simulink model "PC_CONTROL_STATION"  (R2023b)
settings: Solver=FixedStepAuto  StartTime=0.0  StopTime=inf  RelTol=1e-3  EnableMultiTasking=on
InitFcn:
  | if RUN_MODE~=5
  |     % clear rpi;
  |     rpi = raspberrypi(CAR_IP, 'pi', 'LabControl');
  |     stopModel(rpi,'CAR_CONTROL_SYSTEM')
  |     while isModelRunning(rpi,'CAR_CONTROL_SYSTEM')
  |          stopModel(rpi,'CAR_CONTROL_SYSTEM')
  |     end
  |     runModel(rpi,'CAR_CONTROL_SYSTEM')
  |      while isModelRunning(rpi,'CAR_CONTROL_SYSTEM')==false
  |          runModel(rpi,'CAR_CONTROL_SYSTEM')
  |      end
  |      % clear rpi;
  | end
StopFcn:
  | if RUN_MODE~=5
  |    clear rpi;
  |    rpi = raspberrypi(CAR_IP, 'pi', 'LabControl');
  |    stopModel(rpi,'CAR_CONTROL_SYSTEM')
  |    while isModelRunning(rpi,'CAR_CONTROL_SYSTEM')
  |    end
  |    clear rpi;
  | end
model workspace (MAT data in the model file):
  SL_ROS_VariableLengthArrays_MaxSizes.CommonInfo.ArrayTruncateAction = 'EmitWarning'
  SL_ROS_VariableLengthArrays_MaxSizes.MsgTypeMap = containers.Map
  SL_ROS_VariableLengthArrays_MaxSizes.MsgTypeMap.serialization.keys = {'std_msgs/UInt8MultiArray'}
  SL_ROS_VariableLengthArrays_MaxSizes.MsgTypeMap.serialization.values{1}.PropertyName = 'data'
  SL_ROS_VariableLengthArrays_MaxSizes.MsgTypeMap.serialization.values{1}.DataType = 'uint8'
  SL_ROS_VariableLengthArrays_MaxSizes.MsgTypeMap.serialization.values{1}.MaxLength = 1400
  SL_ROS_VariableLengthArrays_MaxSizes.MsgTypeMap.serialization.uniformity = 0
  SL_ROS_VariableLengthArrays_MaxSizes.MsgTypeMap.serialization.keyType = 'char'
  SL_ROS_VariableLengthArrays_MaxSizes.MsgTypeMap.serialization.valueType = 'any'
values from neighbouring files (symbols this model uses):
  data = theClient.GetLastFrameOfData()    [FuncMotive.m]
undefined symbols (not defined in the file or in its folder): CONTROL, CONTROL_INI, data_SL_Info, MD25, MSG, SAMPLING_TIME, Standard_Devices, SYSID_INPUT, TCP_Protocol, UDP_Protocol
libraries: simulink x51, sldrtlib x46, dspsigattribs x7, ros2lib x3, ctrlSharedLib x2, aerolibanimutils x1
(part 1 of 8)
Description:
  | Packet Input/Output
  | 
  | The example model "sldrtex_packetio" shows how to transfer data through
  | UDP communication protocol using binary encoding. The model sends data
  | within one computer, from one UDP port to another. You can modify the
  | model to communicate between two computers by splitting this model
  | into its send and receive parts and running the models on two computers.
  | The yellow blocks are used to send the data, the blue blocks
  | are used to receive the data. Then, please enter the host names or
  | IP addresses of the two computers into the appropriate fields
  | in the Board Setup dialog.
  | 
  | How to run this model in Normal Mode:
  | 
  | 1) Double-click the orange button to switch to Normal Mode if needed.
  | 2) Start the real-time execution using Simulation->Run.
  | 
  | How to run this model in External Mode:
  | 
  | 1) Double-click the orange button to switch to External Mode if needed.
  | 2) Start the real-time execution using Simulation->Run. The model will automatically
  |    build, connect to Simulink in External Mode and start.
settings Model: SimulationMode=external  ExtModeTrigDuration=24000  Creator=The MathWorks, Inc.  LastModifiedBy=diego-ubuntu
settings SolverCC: AlgebraicLoopSolver=TrustRegion
settings DataIOCC: LimitDataPoints=on  SaveFormat=Array  SignalLoggingSaveFormat=ModelDataLogs  ReturnWorkspaceOutputs=off
settings OptimizationCC: EnhancedBackFolding=on  PassReuseOutputArgsThreshold=0  ExpressionDepthLimit=2147483647  InitFltsAndDblsToZero=on  EfficientMapNaN2IntZero=off  MaxStackSize=64  OptimizeBlockOrder=speed  DifferentSizesBufferReuse=on  OptimizationCustomize=off
settings DebuggingCC: MergeDetectMultiDrivingBlocksExec=none  SolverPrmCheckMsg=warning  ParameterTunabilityLossMsg=error  FcnCallInpInsideContextMsg=warning  UnconnectedInputMsg=warning  UnconnectedOutputMsg=warning  UnconnectedLineMsg=warning  AllowSymbolicDim=off  StateNameClashWarn=warning  SFUnexpectedBacktrackingDiag=warning  SFNoUnconditionalDefaultTransitionDiag=warning  SFExecutionAtInitializationDiag=none  ArithmeticOperatorsInVariantConditions=warning
settings HardwareCC: ProdBitPerLong=64  ProdHWDeviceType=Intel->x86-64 (Linux 64)
settings ModelReferenceCC: EnableRefExpFcnMdlSchedulingChecks=on  PropagateSignalLabelsOutOfModel=off
settings SFSimCC: SimUseLocalCustomCode=off  MATLABDynamicMemAlloc=off  CustomCodeUndefinedFunction=UseInterfaceOnly
settings RTWCC: Description=Simulink Desktop Real-Time  SystemTargetFile=sldrt.tlc  TemplateMakefile=sldrt.tmf  RTWUseLocalCustomCode=off  Toolchain=Colcon Tools  RTWCompilerOptimization=on  DLArmComputeVersion=19.05
settings CodeAppCC: ForceParamTrailComments=on  MaxIdLength=95  OperatorAnnotations=on
settings SimulinkDesktopRealTimeCC: TargetLibSuffix=_sldrt.a  TargetPreCompLibLocation=/usr/local/MATLAB/R2023b/toolbox/sldrt/lib/glnxa64  TargetLangStandard=C89/C90 (ANSI)
settings ConfigComp: CovMetricSettings=dsw  CovSaveCumulativeToWorkspaceVar=on  CovSaveSingleToWorkspaceVar=on  CovExternalEMLEnable=off

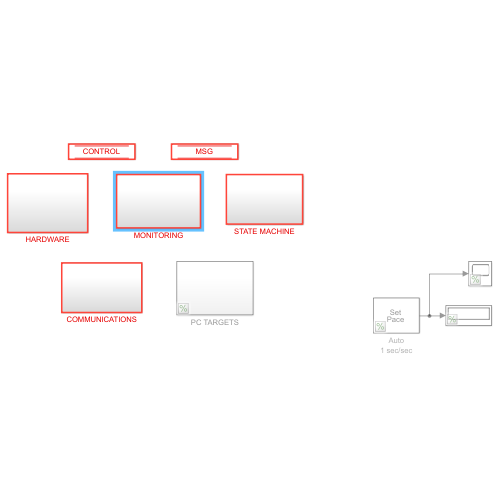
[thumbnail: Simulink's stored preview of the top-level diagram]
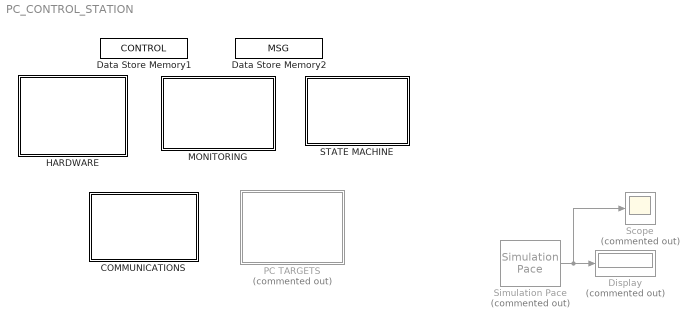
== system PC_CONTROL_STATION ==
  COMMUNICATIONS : Subsystem  Priority=40
      settings: RTWSystemCode=Nonreusable function  RTWFcnNameOpts=Use subsystem name  RTWFileNameOpts=Use subsystem name  FunctionWithSeparateData=on
  Data Store Memory1 : DataStoreMemory  Priority=2  DataStoreName=CONTROL  ReadBeforeWriteMsg=warning  WriteAfterWriteMsg=warning  WriteAfterReadMsg=warning  InitialValue=CONTROL_INI  ShowAdditionalParam=off  OutDataTypeStr=Bus: CONTROL_Bus
  Data Store Memory2 : DataStoreMemory  Priority=2  DataStoreName=MSG  ReadBeforeWriteMsg=warning  WriteAfterWriteMsg=warning  WriteAfterReadMsg=warning  InitialValue=MSG_INI  ShowAdditionalParam=off  OutDataTypeStr=Bus: MSG_Bus
  Display : Display  Commented=on
  HARDWARE : Subsystem  Priority=50  SystemSampleTime=SAMPLING_TIME
      settings: RTWSystemCode=Nonreusable function  RTWFcnNameOpts=Use subsystem name  RTWFileNameOpts=Use subsystem name  FunctionWithSeparateData=on
  MONITORING : Subsystem  Priority=1000
  PC TARGETS : Subsystem  Priority=5  Commented=on
  STATE MACHINE : Subsystem
  Scope : Scope  Commented=on
  Simulation Pace : aerolibanimutils/Simulation Pace  Commented=on  SimulationPace=1  SleepMode=Auto  OutputPaceError=on  SampleTime=CONTROL_INI.PARAM.COMM_SAMPLING_TIME
  wires:
  Simulation Pace/1 -> Scope/1, Display/1

== system PC_CONTROL_STATION/COMMUNICATIONS ==
  Compare To Zero1 : simulink/Logic and Bit Operations/Compare To Zero  relop=>  OutDataTypeStr=boolean
  Compare To Zero2 : simulink/Logic and Bit Operations/Compare To Zero  relop=>  OutDataTypeStr=boolean
  Compare To Zero3 : simulink/Logic and Bit Operations/Compare To Zero  relop=>  OutDataTypeStr=boolean
  Data Store Read1 : DataStoreRead  DataStoreName=MSG  SampleTime=CONTROL_INI.PARAM.COMM_SAMPLING_TIME  DataStoreElements=MSG.RX_BUFFER(1,1)  IndexOptions=Index vector (dialog)  Indices=1  OutputSizes=1
  Data Store Read2 : DataStoreRead  DataStoreName=CONTROL  DataStoreElements=CONTROL.STATE.CURRENT_STATUS_PC  IndexOptions=Index vector (dialog)  Indices=1  OutputSizes=1
  Data Store Read3 : DataStoreRead  DataStoreName=MSG  SampleTime=CONTROL_INI.PARAM.COMM_SAMPLING_TIME  DataStoreElements=MSG.TX_ID(1,1)  IndexOptions=Index vector (dialog)  Indices=1  OutputSizes=1
  Display1 : Display
  Display2 : Display
  Logical Operator1 : Logic  AllPortsSameDT=off  OutDataTypeStr=boolean
  MSG_RX : Subsystem  Priority=10
      settings: RTWSystemCode=Nonreusable function  FunctionWithSeparateData=on
  "MSG_TX " : Subsystem  Priority=10
      settings: RTWSystemCode=Nonreusable function  FunctionWithSeparateData=on
  wires:
  Data Store Read1/1 -> Compare To Zero1/1
  Data Store Read3/1 -> Compare To Zero2/1
  Compare To Zero2/1 -> "MSG_TX "/Enable, Display1/1
  Logical Operator1/1 -> MSG_RX/Enable, Display2/1
  Data Store Read2/1 -> Compare To Zero3/1
  Compare To Zero1/1 -> Logical Operator1/1
  Compare To Zero3/1 -> Logical Operator1/2

== system PC_CONTROL_STATION/HARDWARE ==
  ROS2_MONITORING : Subsystem
  RT_MONITORING : Subsystem  Commented=on

== system PC_CONTROL_STATION/MONITORING ==
  ADAPTIVE CONTROL STR : Subsystem  Commented=on
  FV COMPETITION: SCOPES : Subsystem  Commented=on  TreatAsAtomicUnit=on
      settings: MinAlgLoopOccurrences=on
  HARDWARE: SCOPES : Subsystem  Priority=1000  Commented=on
  NAV COMPETITION: SCOPES : Subsystem  Priority=20  Commented=on  TreatAsAtomicUnit=on
      settings: MinAlgLoopOccurrences=on
  PC: SCOPES : Subsystem
  SYSTEM IDENTIFICATION : Subsystem  Commented=on
      mask init:
      | %%%%%%%%%%%%%%%%%%%%%%%%%%%%%%%%%%%%%%%%%%%%%%%%%%%%%%
      | %%  STATE VARIABLE FILTER FOR SYSTEM IDENTIFICATION  %
      | %%%%%%%%%%%%%%%%%%%%%%%%%%%%%%%%%%%%%%%%%%%%%%%%%%%%%%
      | % Natural frequency (rad/s)
      | SVF_FREQ = 10;
      | % Factor defining band pass width
      | SVF_FACTOR = 5;
      | % FILTER ORDER/2
      | SVF_ORD = 2;
      | % Km/(Tm*Tf*s^2 + (Tm+Tf)*s + 1) = Km/Tm/Tf/(s^2 + (Tm+Tf)/Tm/Tf*s + 1/Tm/Tf)
      | % b0/(s^2 + a1*s + a0)
      | % D2y + a1*D1y + a0*y = b0*u
      | % D1y + a1*y + a0*I1y = b0*I1u
      | % D1yf = - a1*yf - a0*I1y + b0I1uf
      | %  -a1=-(Tm+Tf)/Tm/Tf / -a0=-1/Tm/Tf / b0=Km/Tm/Tf 
      | % Butterworh filter desig
      | [SVF_NUM,SVF_DEN]=butter(SVF_ORD,[SVF_FREQ/SVF_FACTOR SVF_FACTOR*SVF_FREQ],'s');
      | % Controlability canonical-form 
      | SVF_A = single([zeros(2*SVF_ORD-1,1) eye(2*SVF_ORD-1) ; -SVF_DEN(end:-1:2)]);
      | SVF_B = single([zeros(2*SVF_ORD-1,1) ; SVF_NUM(end-SVF_ORD)]);
      | % Sampling time
      | ts = 10e-3;
      | % Triangular hold
      | % x[k] = Ad*x[k-1] + B1d*u[k-1] + B2d*u[k]
      | % Ad = expm(A*ts)
      | % B1d = A\(Ad+inv(A)/ts-inv(A)*Ad/ts)*B;
      | % B2d = A\(inv(A)*Ad/ts-eye(2)-inv(A)/ts)*B;
      | SVF_Ad = expm(SVF_A*ts);
      | SVF_B1d = SVF_A\(SVF_Ad+inv(SVF_A)/ts-SVF_A\SVF_Ad/ts)*SVF_B;
      | SVF_B2d = SVF_A\(SVF_A\SVF_Ad/ts-eye(2*SVF_ORD)-inv(SVF_A)/ts)*SVF_B;

== system PC_CONTROL_STATION/PC TARGETS ==
  Compare To Constant4 : simulink/Logic and Bit Operations/Compare To Constant  relop=>  const=0  OutDataTypeStr=boolean
  Data Store Read9 : DataStoreRead  DataStoreName=CONTROL  SampleTime=SAMPLING_TIME  DataStoreElements=CONTROL.STATE.CONTROL_STATUS  IndexOptions=Index vector (dialog)  Indices=1  OutputSizes=1
  PC TARGETS : Subsystem  Priority=5  Commented=on  TreatAsAtomicUnit=on
      settings: MinAlgLoopOccurrences=on
  wires:
  Data Store Read9/1 -> Compare To Constant4/1
  Compare To Constant4/1 -> PC TARGETS/Enable

== system PC_CONTROL_STATION/STATE MACHINE ==
  Data Store Read2 : DataStoreRead  DataStoreName=MSG  SampleTime=CONTROL_INI.PARAM.COMM_SAMPLING_TIME  IndexOptions=Index vector (dialog)  Indices=1  OutputSizes=1
  Data Store Read7 : DataStoreRead  DataStoreName=CONTROL  SampleTime=CONTROL_INI.PARAM.COMM_SAMPLING_TIME  IndexOptions=Index vector (dialog)  Indices=1  OutputSizes=1
  Data Store Write1 : DataStoreWrite  DataStoreName=MSG  IndexOptions=Index vector (dialog)  Indices=1  OutputSizes=1
  Data Store Write3 : DataStoreWrite  DataStoreName=CONTROL  IndexOptions=Index vector (dialog)  Indices=1  OutputSizes=1
  Display : Display
  STATE MACHINE UPDATE : MATLAB Function  Priority=60  TreatAsAtomicUnit=on
  Scope : Scope
  wires:
  STATE MACHINE UPDATE/1(CONTROL) -> Data Store Write3/1
  Data Store Read7/1 -> STATE MACHINE UPDATE/1(CONTROL_IN)
  Data Store Read2/1 -> STATE MACHINE UPDATE/2(MSG_IN)
  STATE MACHINE UPDATE/2(MSG) -> Data Store Write1/1
  STATE MACHINE UPDATE/3(DATA_DIFF) -> Scope/1, Display/1

== system PC_CONTROL_STATION/COMMUNICATIONS/MSG_RX ==
  Enable : EnablePort
  Data Store Read : DataStoreRead  DataStoreName=MSG  SampleTime=CONTROL_INI.PARAM.COMM_SAMPLING_TIME  IndexOptions=Index vector (dialog)  Indices=1  OutputSizes=1
  Data Store Read2 : DataStoreRead  DataStoreName=CONTROL  SampleTime=CONTROL_INI.PARAM.COMM_SAMPLING_TIME  IndexOptions=Index vector (dialog)  Indices=1  OutputSizes=1
  Data Store Write1 : DataStoreWrite  DataStoreName=MSG  SampleTime=CONTROL_INI.PARAM.COMM_SAMPLING_TIME  IndexOptions=Index vector (dialog)  Indices=1  OutputSizes=1
  Data Store Write2 : DataStoreWrite  DataStoreName=CONTROL  SampleTime=CONTROL_INI.PARAM.COMM_SAMPLING_TIME  IndexOptions=Index vector (dialog)  Indices=1  OutputSizes=1
  MSG DECODER : MATLAB Function  Priority=20  TreatAsAtomicUnit=on
  wires:
  MSG DECODER/1(MSG) -> Data Store Write1/1
  Data Store Read/1 -> MSG DECODER/1(MSG_IN)
  MSG DECODER/2(CONTROL) -> Data Store Write2/1
  Data Store Read2/1 -> MSG DECODER/2(CONTROL_IN)

== system PC_CONTROL_STATION/COMMUNICATIONS/MSG_TX  ==
  Enable : EnablePort
  Data Store Read : DataStoreRead  DataStoreName=MSG  SampleTime=CONTROL_INI.PARAM.COMM_SAMPLING_TIME  IndexOptions=Index vector (dialog)  Indices=1  OutputSizes=1
  Data Store Read6 : DataStoreRead  DataStoreName=CONTROL  SampleTime=CONTROL_INI.PARAM.COMM_SAMPLING_TIME  IndexOptions=Index vector (dialog)  Indices=1  OutputSizes=1
  Data Store Write1 : DataStoreWrite  DataStoreName=MSG  SampleTime=CONTROL_INI.PARAM.COMM_SAMPLING_TIME  IndexOptions=Index vector (dialog)  Indices=1  OutputSizes=1
  MSG CODER : MATLAB Function  Priority=20  TreatAsAtomicUnit=on
  wires:
  Data Store Read/1 -> MSG CODER/1(MSG_IN)
  MSG CODER/1(MSG) -> Data Store Write1/1
  Data Store Read6/1 -> MSG CODER/2(CONTROL)

== system PC_CONTROL_STATION/HARDWARE/ROS2_MONITORING ==
  Compare To Zero : simulink/Logic and Bit Operations/Compare To Zero  relop=>  OutDataTypeStr=boolean
  Data Store Read : DataStoreRead  DataStoreName=MSG  SampleTime=CONTROL_INI.PARAM.COMM_SAMPLING_TIME  DataStoreElements=MSG.TX_BUFFER(1,1)  IndexOptions=Index vector (dialog)  Indices=1  OutputSizes=1
  MSG_RX : Subsystem  Priority=10
      settings: RTWSystemCode=Nonreusable function  FunctionWithSeparateData=on
  "MSG_TX " : Subsystem  Priority=10
      settings: RTWSystemCode=Nonreusable function  FunctionWithSeparateData=on
  wires:
  Compare To Zero/1 -> "MSG_TX "/Enable
  Data Store Read/1 -> Compare To Zero/1

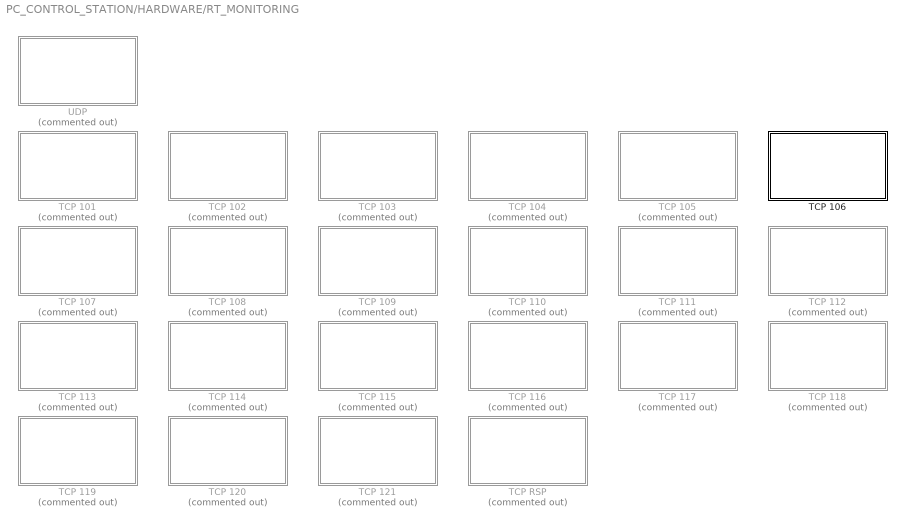
== system PC_CONTROL_STATION/HARDWARE/RT_MONITORING ==
  TCP 101 : Subsystem  Commented=on
  TCP 102 : Subsystem  Commented=on
  TCP 103 : Subsystem  Commented=on
  TCP 104 : Subsystem  Commented=on
  TCP 105 : Subsystem  Commented=on
  TCP 106 : Subsystem
  TCP 107 : Subsystem  Commented=on
  TCP 108 : Subsystem  Commented=on
  TCP 109 : Subsystem  Commented=on
  TCP 110 : Subsystem  Commented=on
  TCP 111 : Subsystem  Commented=on
  TCP 112 : Subsystem  Commented=on
  TCP 113 : Subsystem  Commented=on
  TCP 114 : Subsystem  Commented=on
  TCP 115 : Subsystem  Commented=on
  TCP 116 : Subsystem  Commented=on
  TCP 117 : Subsystem  Commented=on
  TCP 118 : Subsystem  Commented=on
  TCP 119 : Subsystem  Commented=on
  TCP 120 : Subsystem  Commented=on
  TCP 121 : Subsystem  Commented=on
  TCP RSP : Subsystem  Commented=on
  UDP : Subsystem  Commented=on

== system PC_CONTROL_STATION/MONITORING/ADAPTIVE CONTROL STR ==
  Data Store Read : DataStoreRead  DataStoreName=CONTROL  SampleTime=SAMPLING_TIME  DataStoreElements=CONTROL.TARGET.FORWARD_VEL_REF#CONTROL.INPUT.FORWARD_VEL#CONTROL.OUTPUT.MOTOR_VOLT_CD(1,1)#CONTROL.PARAM.VEL_GAIN#CONTROL.PARAM.VEL_GAIN_EST#CONTROL.PARAM.VEL_TIME_CONSTANT#CONTROL.PARAM.VEL_TIME_CONSTANT_EST#CONTROL.PARAM.FILT_TIME_CONSTANT_ACT#CONTROL.PARAM.FILT_TIME_CONSTANT_EST#CONTROL.PARAM.FORWARD_VEL_PID.K#CONTROL.PARAM.FV_PI_STR_K#CONTROL.PARAM.FORWARD_VEL_PID.Ti#CONTROL.PARAM.FV_PI_STR_Ti#CONTROL.PARAM.FORWARD_VEL_PID.b#CONTROL.PARAM.FV_PI_STR_b#CONTROL.PARAM.ADPT_FLAG  IndexOptions=Index vector (dialog)  Indices=1  OutputSizes=1
  Mux{1..7} (7 alike) : Mux  Inputs=2
  SCOPE_STR : Scope  NumInputPorts=9
  wires:
  Mux4/1 -> SCOPE_STR/1
  Data Store Read/1 -> Mux4/1
  Data Store Read/2 -> Mux4/2
  Data Store Read/3 -> SCOPE_STR/2
  Mux1/1 -> SCOPE_STR/3
  Data Store Read/4 -> Mux1/1
  Data Store Read/5 -> Mux1/2
  Mux2/1 -> SCOPE_STR/4
  Data Store Read/6 -> Mux2/1
  Data Store Read/7 -> Mux2/2
  Mux3/1 -> SCOPE_STR/5
  Data Store Read/8 -> Mux3/1
  Data Store Read/9 -> Mux3/2
  Mux5/1 -> SCOPE_STR/6
  Data Store Read/10 -> Mux5/1
  Data Store Read/11 -> Mux5/2
  Data Store Read/12 -> Mux6/1
  Data Store Read/13 -> Mux6/2
  Mux6/1 -> SCOPE_STR/7
  Mux7/1 -> SCOPE_STR/8
  Data Store Read/14 -> Mux7/1
  Data Store Read/15 -> Mux7/2
  Data Store Read/16 -> SCOPE_STR/9

== system PC_CONTROL_STATION/MONITORING/FV COMPETITION: SCOPES ==
  Data Store Read1 : DataStoreRead  DataStoreName=CONTROL  SampleTime=SAMPLING_TIME  DataStoreElements=CONTROL.TARGET.FORWARD_VEL_REF#CONTROL.INPUT.FORWARD_VEL#CONTROL.OUTPUT.MOTOR_VOLT_CD(1,1)#CONTROL.STATE.COMP_IAE  IndexOptions=Index vector (dialog)  Indices=1  OutputSizes=1
  Display : Display
  FV COMPETITION SCOPE: SIM : Scope  NumInputPorts=3
  Mux6 : Mux  Inputs=2
  wires:
  Mux6/1 -> FV COMPETITION SCOPE: SIM/1
  Data Store Read1/1 -> Mux6/1
  Data Store Read1/2 -> Mux6/2
  Data Store Read1/3 -> FV COMPETITION SCOPE: SIM/2
  Data Store Read1/4 -> Display/1, FV COMPETITION SCOPE: SIM/3

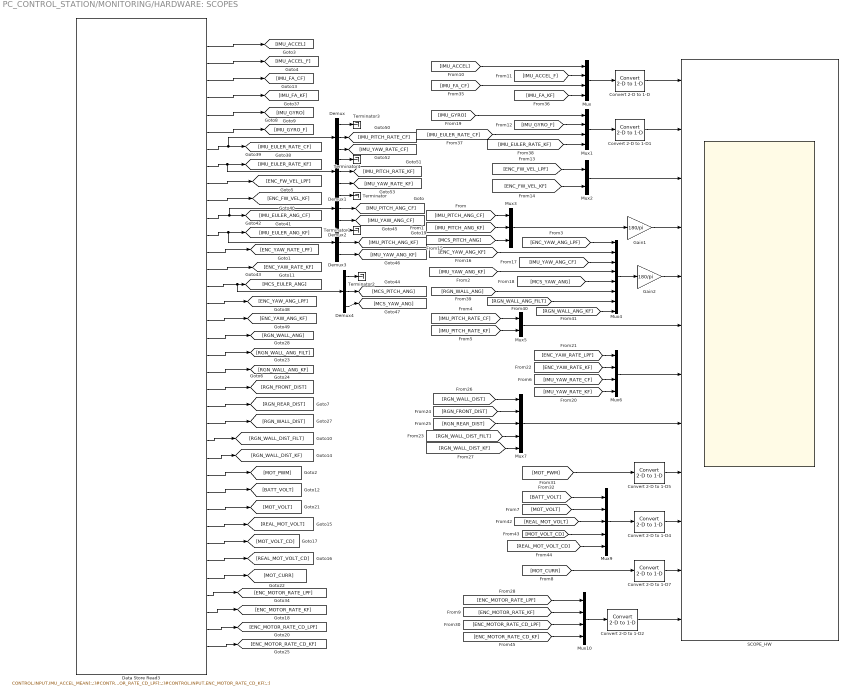
== system PC_CONTROL_STATION/MONITORING/HARDWARE: SCOPES ==
  Convert 2-D to 1-D{,1..2,4..5,7} (6 alike) : dspsigattribs/Convert 2-D to 1-D
  Data Store Read3 : DataStoreRead  DataStoreName=CONTROL  SampleTime=CONTROL_INI.PARAM.COMM_SAMPLING_TIME  DataStoreElements=CONTROL.INPUT.IMU_ACCEL_MEAN(:,:)#CONTROL.INPUT.IMU_ACCEL_MEAN_FILT(:,:)#CONTROL.INPUT.IMU_FORWARD_ACCEL_CF#CONTROL.INPUT.IMU_FORWARD_ACCEL_KF#CONTROL.INPUT.IMU_GYRO_MEAN(:,:)#CONTROL.INPUT.IMU_GYRO_MEAN_FILT(:,:)#CONTROL.INPUT.IMU_EULER_RATE_CF(:,:)#CONTROL.INPUT.IMU_EULER_RATE_KF(:,:)#CONTROL.INPUT.ENC_FORWARD_VEL_LPF#CONTROL.INPUT.ENC_FORWARD_VEL_KF#CONTROL.INPUT.IMU_EULER_ANG_CF(:,:)#CONTROL.INPUT.IMU_EULER_ANG_KF(:,:)#CONTROL.INPUT.ENC_YAW_RATE_LPF#CONTROL.INPUT.ENC_YAW_RATE_KF#CONTROL.INPUT.MCS_EULER_ANG(:,:)#CONTROL.INPUT.ENC_YAW_ANG_LPF#CONTROL.INPUT.ENC_YAW_ANG_KF#CONTROL.INPUT.RANGE_WALL_ANG#CONTROL.INPUT.WALL_ANG_FILT#CONTROL.INPUT.WALL_ANG_KF#CONTROL.INPUT.RANGE_FRONT_DIST#CONTROL.INPUT.RANGE_REAR_DIST#CONTROL.INPUT.RANGE_WALL_DIST#CONTROL.INPUT.WALL_DIST_FILT#CONTROL.INPUT.WALL_DIST_KF#CONTROL.OUTPUT.MOTOR_PWM(:,:)#CONTROL.INPUT.BATTERY_VOLT#CONTROL.OUTPUT.MOTOR_VOLT(:,:)#CONTROL.OUTPUT.REAL_MOTOR_VOLT(:,:)#CONTROL.OUTPUT.MOTOR_VOLT_CD(:,:)#CONTROL.OUTPUT.REAL_MOTOR_VOLT_CD(:,:)#CONTROL.INPUT.MOTOR_CURRENT(:,:)#CONTROL.INPUT.ENC_MOTOR_RATE_LPF(:,:)#CONTROL.INPUT.ENC_MOTOR_RATE_KF(:,:)#CONTROL.INPUT.ENC_MOTOR_RATE_CD_LPF(:,:)#CONTROL.INPUT.ENC_MOTOR_RATE_CD_KF(:,:)  IndexOptions=Index vector (dialog)  Indices=1  OutputSizes=1
  Demux{,1..4} (5 alike) : Demux  Outputs=3
  Gain1 : Gain  Gain=180/pi
  Gain2 : Gain  Gain=180/pi
  Mux{,1,6,10} (4 alike) : Mux
  Mux2 : Mux  Inputs=2
  Mux3 : Mux  Inputs=3
  Mux4 : Mux  Inputs=8
  Mux5 : Mux  Inputs=2
  Mux7 : Mux  Inputs=5
  Mux9 : Mux  Inputs=5
  SCOPE_HW : Scope  NumInputPorts=12
  Terminator{,1..4} (5 alike) : Terminator
  wires:
  [MOT_CURR] -> Convert 2-D to 1-D7/1
  Convert 2-D to 1-D/1 -> SCOPE_HW/1
  Convert 2-D to 1-D1/1 -> SCOPE_HW/2
  Mux2/1 -> SCOPE_HW/3
  [IMU_ACCEL] -> Mux/1
  Mux/1 -> Convert 2-D to 1-D/1
  [IMU_ACCEL_F] -> Mux/2
  [ENC_FW_VEL_LPF] -> Mux2/1
  [ENC_FW_VEL_KF] -> Mux2/2
  [IMU_PITCH_ANG_CF] -> Mux3/1
  [IMU_PITCH_ANG_KF] -> Mux3/2
  Mux3/1 -> Gain1/1
  Gain1/1 -> SCOPE_HW/4
  Mux4/1 -> Gain2/1
  Gain2/1 -> SCOPE_HW/5
  Mux5/1 -> SCOPE_HW/6
  [IMU_PITCH_RATE_CF] -> Mux5/1
  [IMU_PITCH_RATE_KF] -> Mux5/2
  Mux6/1 -> SCOPE_HW/7
  Mux7/1 -> SCOPE_HW/8
  [RGN_WALL_DIST] -> Mux7/1
  [RGN_FRONT_DIST] -> Mux7/2
  [RGN_REAR_DIST] -> Mux7/3
  Mux9/1 -> Convert 2-D to 1-D4/1
  [MOT_VOLT] -> Mux9/2
  [BATT_VOLT] -> Mux9/1
  [MOT_PWM] -> Convert 2-D to 1-D5/1
  Convert 2-D to 1-D5/1 -> SCOPE_HW/9
  Convert 2-D to 1-D4/1 -> SCOPE_HW/10
  Convert 2-D to 1-D7/1 -> SCOPE_HW/11
  Data Store Read3/1 -> [IMU_ACCEL]
  Data Store Read3/2 -> [IMU_ACCEL_F]
  [ENC_MOTOR_RATE_KF] -> Mux10/2
  Mux10/1 -> Convert 2-D to 1-D2/1
  [ENC_MOTOR_RATE_LPF] -> Mux10/1
  Data Store Read3/32 -> [MOT_CURR]
  Data Store Read3/33 -> [ENC_MOTOR_RATE_LPF]
  Data Store Read3/34 -> [ENC_MOTOR_RATE_KF]
  Data Store Read3/5 -> [IMU_GYRO]
  Data Store Read3/6 -> [IMU_GYRO_F]
  Data Store Read3/3 -> [IMU_FA_CF]
  Data Store Read3/4 -> [IMU_FA_KF]
  [IMU_FA_CF] -> Mux/3
  [IMU_FA_KF] -> Mux/4
  Data Store Read3/7 -> Demux/1, [IMU_EULER_RATE_CF]
  Data Store Read3/8 -> Demux1/1, [IMU_EULER_RATE_KF]
  Mux1/1 -> Convert 2-D to 1-D1/1
  [IMU_GYRO] -> Mux1/1
  [IMU_GYRO_F] -> Mux1/2
  [IMU_EULER_RATE_CF] -> Mux1/3
  [IMU_EULER_RATE_KF] -> Mux1/4
  Data Store Read3/9 -> [ENC_FW_VEL_LPF]
  Data Store Read3/10 -> [ENC_FW_VEL_KF]
  Data Store Read3/11 -> Demux2/1, [IMU_EULER_ANG_CF]
  Data Store Read3/12 -> Demux3/1, [IMU_EULER_ANG_KF]
  Demux2/2 -> [IMU_PITCH_ANG_CF]
  Demux3/2 -> [IMU_PITCH_ANG_KF]
  Demux4/2 -> [MCS_PITCH_ANG]
  [MCS_PITCH_ANG] -> Mux3/3
  Demux2/3 -> [IMU_YAW_ANG_CF]
  Demux3/3 -> [IMU_YAW_ANG_KF]
  Demux2/1 -> Terminator/1
  Demux3/1 -> Terminator1/1
  Demux4/3 -> [MCS_YAW_ANG]
  Demux4/1 -> Terminator2/1
  [ENC_YAW_ANG_LPF] -> Mux4/1
  [ENC_YAW_ANG_KF] -> Mux4/2
  [IMU_YAW_ANG_CF] -> Mux4/3
  [IMU_YAW_ANG_KF] -> Mux4/4
  [MCS_YAW_ANG] -> Mux4/5
  [RGN_WALL_ANG] -> Mux4/6
  [RGN_WALL_ANG_FILT] -> Mux4/7
  [RGN_WALL_ANG_KF] -> Mux4/8
  Demux/2 -> [IMU_PITCH_RATE_CF]
  Demux1/2 -> [IMU_PITCH_RATE_KF]
  Demux/1 -> Terminator3/1
  Demux1/1 -> Terminator4/1
  Demux/3 -> [IMU_YAW_RATE_CF]
  Demux1/3 -> [IMU_YAW_RATE_KF]
  Data Store Read3/14 -> [ENC_YAW_RATE_KF]
  Data Store Read3/15 -> Demux4/1, [MCS_EULER_ANG]
  Data Store Read3/16 -> [ENC_YAW_ANG_LPF]
  Data Store Read3/17 -> [ENC_YAW_ANG_KF]
  Data Store Read3/18 -> [RGN_WALL_ANG]
  Data Store Read3/19 -> [RGN_WALL_ANG_FILT]
  Data Store Read3/20 -> [RGN_WALL_ANG_KF]
  Data Store Read3/13 -> [ENC_YAW_RATE_LPF]
  Data Store Read3/21 -> [RGN_FRONT_DIST]
  Data Store Read3/22 -> [RGN_REAR_DIST]
  Data Store Read3/23 -> [RGN_WALL_DIST]
  Data Store Read3/24 -> [RGN_WALL_DIST_FILT]
  Data Store Read3/25 -> [RGN_WALL_DIST_KF]
  [RGN_WALL_DIST_FILT] -> Mux7/4
  [RGN_WALL_DIST_KF] -> Mux7/5
  Data Store Read3/26 -> [MOT_PWM]
  Data Store Read3/27 -> [BATT_VOLT]
  Data Store Read3/28 -> [MOT_VOLT]
  Data Store Read3/29 -> [REAL_MOT_VOLT]
  Data Store Read3/31 -> [REAL_MOT_VOLT_CD]
  Data Store Read3/30 -> [MOT_VOLT_CD]
  [REAL_MOT_VOLT_CD] -> Mux9/5
  [REAL_MOT_VOLT] -> Mux9/3
  [MOT_VOLT_CD] -> Mux9/4
  Data Store Read3/35 -> [ENC_MOTOR_RATE_CD_LPF]
  Data Store Read3/36 -> [ENC_MOTOR_RATE_CD_KF]
  [ENC_MOTOR_RATE_CD_LPF] -> Mux10/3
  [ENC_MOTOR_RATE_CD_KF] -> Mux10/4
  Convert 2-D to 1-D2/1 -> SCOPE_HW/12
  [IMU_YAW_RATE_CF] -> Mux6/3
  [IMU_YAW_RATE_KF] -> Mux6/4
  [ENC_YAW_RATE_LPF] -> Mux6/1
  [ENC_YAW_RATE_KF] -> Mux6/2

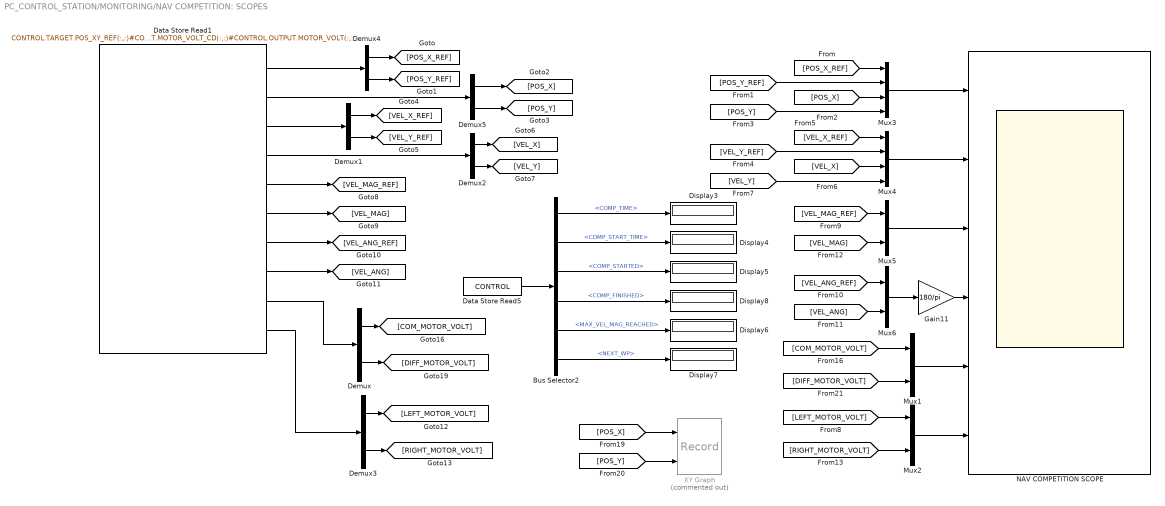
== system PC_CONTROL_STATION/MONITORING/NAV COMPETITION: SCOPES ==
  Bus Selector2 : BusSelector  OutputSignals=STATE.COMP_TIME,STATE.COMP_START_TIME,STATE.COMP_STARTED,STATE.COMP_FINISHED,STATE.MAX_VEL_MAG_REACHED,STATE.NEXT_WP
  Data Store Read1 : DataStoreRead  DataStoreName=CONTROL  SampleTime=SAMPLING_TIME  DataStoreElements=CONTROL.TARGET.POS_XY_REF(:,:)#CONTROL.INPUT.EARTH_POS(1:2,1)#CONTROL.TARGET.VEL_XY_REF(:,:)#CONTROL.INPUT.EARTH_VEL(1:2,1)#CONTROL.TARGET.NAV_REF(1,1)#CONTROL.INPUT.NAV_MO(1,1)#CONTROL.TARGET.NAV_REF(2,1)#CONTROL.INPUT.NAV_MO(2,1)#CONTROL.OUTPUT.MOTOR_VOLT_CD(:,:)#CONTROL.OUTPUT.MOTOR_VOLT(:,:)  IndexOptions=Index vector (dialog)  Indices=1  OutputSizes=1
  Data Store Read5 : DataStoreRead  DataStoreName=CONTROL  SampleTime=SAMPLING_TIME  IndexOptions=Index vector (dialog)  Indices=1  OutputSizes=1
  Demux{,1..5} (6 alike) : Demux  Outputs=2
  Display{3..8} (6 alike) : Display
  Gain11 : Gain  Gain=180/pi
  Mux{1..2,5..6} (4 alike) : Mux  Inputs=2
  Mux3 : Mux
  Mux4 : Mux
  NAV COMPETITION SCOPE : Scope  NumInputPorts=6
  XY Graph : Record  Commented=on  FileSettingsInternal="{\"entries\":[{\"content\":{\"excelSettings\":{\"content\":{},\"type\":\"Streamout.ExcelSettings\"}},\"type\":\"Streamout.FileSettingStorage\",\"uuid\":\"\"}],\"packageUris\":[\"http:\\/\\/schema.mathworks.com\\/mf0\\/streamout_blocks\\/R2020a\"],\"version\":\"1.0\"}"  Layout=[1 1]  SignalsInternal="{\"entries\":[{\"content\":{\"signals\":[{\"content\":{\"blockPath\":[],\"dimensions\":[1],\"domain\":\"\",\"lineColor\":\"#a2142f\",\"plots\":[ 1 ],\"port\":1,\"signalID\":1,\"signalName\":\"XY Graph:1\"},\"type\":\"RecordBlkView.Signal\",\"uuid\":\"\"},{\"content\":{\"blockPath\":[],\"dimensions\":[1],\"domain\":\"\",\"lineColor\":\"#139fff\",\"plots\":[ 1 ],\"port\":2,\"signalID\":2,\"signalName\":\"XY Graph:2\"},\"type\":\"RecordBlkView.Signal\",\"uuid\":\"\"}]},\"type\":\"RecordBlkView.InputSignals\",\"uuid\":\"\"}],\"packageUris\":[\"http:\\/\\/schema.mathworks.com\\/mf0\\/streamout_blocks\\/R2020a\"],\"version\":\"1.0\"}"  VisualizationBindings="{\"xyplotplugin\":{\"info\":[{\"series\":[{\"bindingParametersList\":[{\"parameter\":\"X-Axis\",\"signalID\":1,\"signalName\":\"XY Graph:1\"},{\"parameter\":\"Y-Axis\",\"signalID\":2,\"signalName\":\"XY Graph:2\"}],\"seriesID\":0}],\"subplotID\":1}]}}"  CompatibilityTag=XY  st=SAMPLING_TIME
  wires:
  Bus Selector2/1 -> Display3/1  "<COMP_TIME>"
  Bus Selector2/4 -> Display8/1  "<COMP_FINISHED>"
  Bus Selector2/3 -> Display5/1  "<COMP_STARTED>"
  Bus Selector2/2 -> Display4/1  "<COMP_START_TIME>"
  Bus Selector2/6 -> Display7/1  "<NEXT_WP>"
  Mux4/1 -> NAV COMPETITION SCOPE/2
  Bus Selector2/5 -> Display6/1  "<MAX_VEL_MAG_REACHED>"
  Gain11/1 -> NAV COMPETITION SCOPE/4
  Mux3/1 -> NAV COMPETITION SCOPE/1
  Mux6/1 -> Gain11/1
  Mux5/1 -> NAV COMPETITION SCOPE/3
  Data Store Read5/1 -> Bus Selector2/1
  Demux4/1 -> [POS_X_REF]
  Demux4/2 -> [POS_Y_REF]
  Demux5/1 -> [POS_X]
  Demux5/2 -> [POS_Y]
  [POS_X_REF] -> Mux3/1
  [VEL_X_REF] -> Mux4/1
  [VEL_Y] -> Mux4/4
  [VEL_MAG_REF] -> Mux5/1
  [VEL_MAG] -> Mux5/2
  [VEL_ANG_REF] -> Mux6/1
  [VEL_ANG] -> Mux6/2
  Data Store Read1/9 -> Demux/1
  [POS_X] -> XY Graph/1
  [POS_Y] -> XY Graph/2
  Demux1/1 -> [VEL_X_REF]
  Demux1/2 -> [VEL_Y_REF]
  Demux2/2 -> [VEL_Y]
  Demux2/1 -> [VEL_X]
  Data Store Read1/1 -> Demux4/1
  Data Store Read1/2 -> Demux5/1
  Data Store Read1/3 -> Demux1/1
  Data Store Read1/4 -> Demux2/1
  Data Store Read1/5 -> [VEL_MAG_REF]
  Data Store Read1/6 -> [VEL_MAG]
  Data Store Read1/7 -> [VEL_ANG_REF]
  Data Store Read1/8 -> [VEL_ANG]
  Demux/1 -> [COM_MOTOR_VOLT]
  Demux/2 -> [DIFF_MOTOR_VOLT]
  [COM_MOTOR_VOLT] -> Mux1/1
  [DIFF_MOTOR_VOLT] -> Mux1/2
  Mux1/1 -> NAV COMPETITION SCOPE/5
  Mux2/1 -> NAV COMPETITION SCOPE/6
  [RIGHT_MOTOR_VOLT] -> Mux2/2
  [LEFT_MOTOR_VOLT] -> Mux2/1
  Data Store Read1/10 -> Demux3/1
  Demux3/1 -> [LEFT_MOTOR_VOLT]
  Demux3/2 -> [RIGHT_MOTOR_VOLT]
  [POS_Y_REF] -> Mux3/2
  [POS_X] -> Mux3/3
  [POS_Y] -> Mux3/4
  [VEL_Y_REF] -> Mux4/2
  [VEL_X] -> Mux4/3

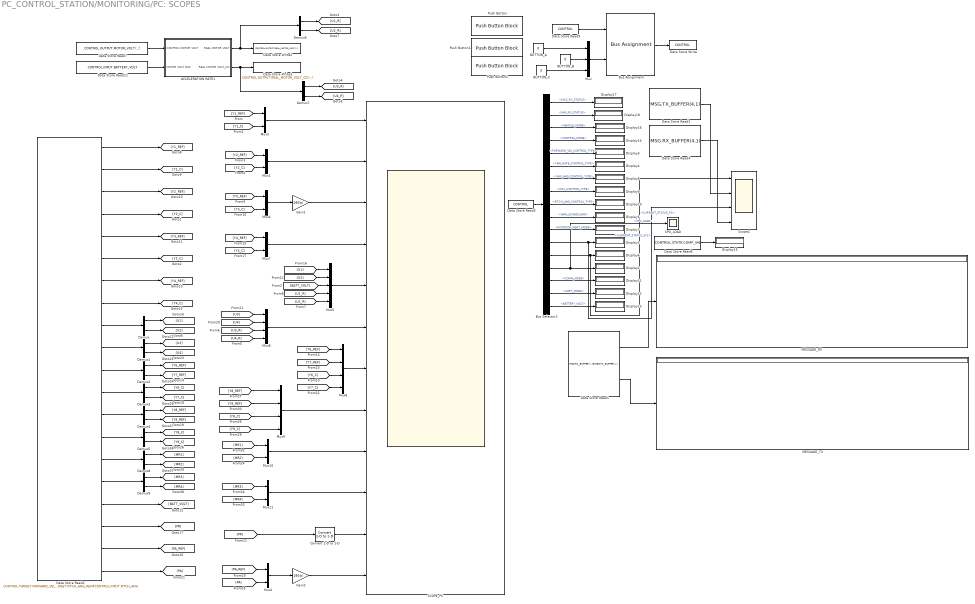
== system PC_CONTROL_STATION/MONITORING/PC: SCOPES ==
  ACCELERATION RATE1 : Subsystem  Priority=50  TreatAsAtomicUnit=on
      settings: MinAlgLoopOccurrences=on
  BUTTON_A : Constant  Value=0  OutDataTypeStr=uint8  SampleTime=CONTROL_INI.PARAM.COMM_SAMPLING_TIME
  BUTTON_B : Constant  Value=0  OutDataTypeStr=uint8  SampleTime=CONTROL_INI.PARAM.COMM_SAMPLING_TIME
  BUTTON_C : Constant  Value=0  OutDataTypeStr=uint8  SampleTime=CONTROL_INI.PARAM.COMM_SAMPLING_TIME
  Bus Assignment : BusAssignment  Priority=40  AssignedSignals=STATE.PC_BUTTONS
  Bus Selector2 : BusSelector  OutputSignals=STATE.MCS_RX_STATUS,STATE.NAV_RX_STATUS,STATE.VEHICLE_MODE,STATE.CONTROL_MODE,STATE.FORWARD_VEL_CONTROL_TYPE,STATE.YAW_RATE_CONTROL_TYPE,STATE.YAW_ANG_CONTROL_TYPE,STATE.WFL_CONTROL_TYPE,STATE.PITCH_ANG_CONTROL_TYPE,STATE.GAIN_SCHEDULING,STATE.ROTATION_MSRT_MODE,STATE.CURRENT_STATUS_SYS,STATE.CURRENT_STATUS_PC,STATE.CPU_LOAD,STATE.COMM_MODE,STATE.UART_MODE,INPUT.BATTERY_VOLT
  CPU_LOAD : Scope
  Convert 2-D to 1-D : dspsigattribs/Convert 2-D to 1-D
  Data Store Read1 : DataStoreRead  DataStoreName=MSG  SampleTime=CONTROL_INI.PARAM.COMM_SAMPLING_TIME  DataStoreElements=MSG.RX_BUFFER(:,:)#MSG.TX_BUFFER(:,:)  IndexOptions=Index vector (dialog)  Indices=1  OutputSizes=1
  Data Store Read11 : DataStoreRead  DataStoreName=CONTROL  SampleTime=CONTROL_INI.PARAM.COMM_SAMPLING_TIME  DataStoreElements=CONTROL.INPUT.BATTERY_VOLT  IndexOptions=Index vector (dialog)  Indices=1  OutputSizes=1
  Data Store Read2 : DataStoreRead  DataStoreName=CONTROL  SampleTime=CONTROL_INI.PARAM.COMM_SAMPLING_TIME  DataStoreElements=CONTROL.TARGET.FORWARD_VEL_REF#CONTROL.INPUT.FORWARD_VEL#CONTROL.TARGET.YAW_RATE_REF#CONTROL.INPUT.YAW_RATE#CONTROL.TARGET.YAW_ANG_REF#CONTROL.INPUT.YAW_ANG#CONTROL.TARGET.WALL_DIST_REF#CONTROL.INPUT.WALL_DIST#CONTROL.OUTPUT.MOTOR_VOLT(:,:)#CONTROL.OUTPUT.MOTOR_VOLT_CD(:,:)#CONTROL.TARGET.POS_XY_REF(:,:)#CONTROL.INPUT.EARTH_POS(1:2,1)#CONTROL.TARGET.VEL_XY_REF(:,:)#CONTROL.INPUT.EARTH_VEL(1:2,1)#CONTROL.INPUT.MOTOR_RATE(:,:)#CONTROL.INPUT.MOTOR_RATE_CD(:,:)#CONTROL.INPUT.BATTERY_VOLT#CONTROL.INPUT.PITCH_RATE#CONTROL.TARGET.PITCH_ANG_REF#CONTROL.INPUT.PITCH_ANG  IndexOptions=Index vector (dialog)  Indices=1  OutputSizes=1
  Data Store Read3 : DataStoreRead  DataStoreName=MSG  SampleTime=CONTROL_INI.PARAM.COMM_SAMPLING_TIME  DataStoreElements=MSG.TX_BUFFER(4,1)  IndexOptions=Index vector (dialog)  Indices=1  OutputSizes=1
  Data Store Read4 : DataStoreRead  DataStoreName=MSG  SampleTime=CONTROL_INI.PARAM.COMM_SAMPLING_TIME  DataStoreElements=MSG.RX_BUFFER(4,1)  IndexOptions=Index vector (dialog)  Indices=1  OutputSizes=1
  Data Store Read5 : DataStoreRead  DataStoreName=CONTROL  SampleTime=CONTROL_INI.PARAM.COMM_SAMPLING_TIME  IndexOptions=Index vector (dialog)  Indices=1  OutputSizes=1
  Data Store Read6 : DataStoreRead  DataStoreName=CONTROL  SampleTime=CONTROL_INI.PARAM.COMM_SAMPLING_TIME  DataStoreElements=CONTROL.STATE.COMP_IAE  IndexOptions=Index vector (dialog)  Indices=1  OutputSizes=1
  Data Store Read7 : DataStoreRead  DataStoreName=CONTROL  SampleTime=CONTROL_INI.PARAM.COMM_SAMPLING_TIME  DataStoreElements=CONTROL.OUTPUT.MOTOR_VOLT(:,:)  IndexOptions=Index vector (dialog)  Indices=1  OutputSizes=1
  Data Store Read9 : DataStoreRead  DataStoreName=CONTROL  SampleTime=CONTROL_INI.PARAM.COMM_SAMPLING_TIME  IndexOptions=Index vector (dialog)  Indices=1  OutputSizes=1
  Data Store Write : DataStoreWrite  DataStoreName=CONTROL  IndexOptions=Index vector (dialog)  Indices=1  OutputSizes=1
  Data Store Write2 : DataStoreWrite  DataStoreName=CONTROL  DataStoreElements=CONTROL.OUTPUT.REAL_MOTOR_VOLT(:,:)  IndexOptions=Index vector (dialog)  Indices=1  OutputSizes=1
  Data Store Write3 : DataStoreWrite  DataStoreName=CONTROL  DataStoreElements=CONTROL.OUTPUT.REAL_MOTOR_VOLT_CD(:,:)  IndexOptions=Index vector (dialog)  Indices=1  OutputSizes=1
  Demux{,1..9} (10 alike) : Demux  Outputs=2
  Display{1..18} (18 alike) : Display
  Gain1 : Gain  Gain=180/pi
  Gain2 : Gain  Gain=180/pi
  MESSAGE_RX : Display
  MESSAGE_TX : Display
  Mux : Mux  Inputs=3
  Mux{1..4,7,10..11} (7 alike) : Mux  Inputs=2
  Mux5 : Mux  Inputs=5
  Mux6 : Mux
  Mux8 : Mux
  Mux9 : Mux
  Push Button : PushButtonBlock  ButtonText=BUTTON A  OffValue=0.000000
  Push Button1 : PushButtonBlock  ButtonText=BUTTON B  OffValue=0.000000
  Push Button2 : PushButtonBlock  ButtonText=BUTTON C  OffValue=0.000000
  SCOPE_PC : Scope  NumInputPorts=12
  Scope2 : Scope  NumInputPorts=4
  wires:
  Data Store Read5/1 -> Bus Selector2/1
  Bus Selector2/11 -> Display7/1  "<ROTATION_MSRT_MODE>"
  Data Store Read1/1 -> MESSAGE_RX/1
  Bus Selector2/10 -> Display5/1  "<GAIN_SCHEDULING>"
  Bus Selector2/12 -> Display1/1, Scope2/3  "<CURRENT_STATUS_SYS>"
  Bus Selector2/14 -> CPU_LOAD/1, Display2/1  "<CPU_LOAD>"
  Data Store Read1/2 -> MESSAGE_TX/1
  Mux/1 -> Bus Assignment/2
  Data Store Read9/1 -> Bus Assignment/1
  Bus Assignment/1 -> Data Store Write/1
  BUTTON_C/1 -> Mux/3
  BUTTON_B/1 -> Mux/2
  BUTTON_A/1 -> Mux/1
  Bus Selector2/13 -> Scope2/1, Display6/1  "<CURRENT_STATUS_PC>"
  Data Store Read3/1 -> Scope2/2
  Data Store Read4/1 -> Scope2/4
  Demux8/2 -> [MR2]
  Demux9/1 -> [MR3]
  Data Store Read2/16 -> Demux9/1
  Data Store Read2/15 -> Demux8/1
  Data Store Read2/2 -> [Y1_C]
  Data Store Read2/7 -> [Y4_REF]
  Demux4/1 -> [Y8_REF]
  Demux5/1 -> [Y8_C]
  Demux3/1 -> [Y6_C]
  Demux2/1 -> [Y6_REF]
  Demux1/1 -> [U3]
  Demux3/2 -> [Y7_C]
  Demux5/2 -> [Y9_C]
  Demux4/2 -> [Y9_REF]
  Demux2/2 -> [Y7_REF]
  Data Store Read2/5 -> [Y3_REF]
  Demux/2 -> [U2]
  Data Store Read2/1 -> [Y1_REF]
  Demux1/2 -> [U4]
  Demux8/1 -> [MR1]
  Data Store Read2/4 -> [Y2_C]
  Data Store Read2/6 -> [Y3_C]
  Demux9/2 -> [MR4]
  Data Store Read2/3 -> [Y2_REF]
  Data Store Read2/8 -> [Y4_C]
  Demux/1 -> [U1]
  [MR1] -> Mux10/1
  [MR4] -> Mux11/2
  Gain1/1 -> SCOPE_PC/3
  Mux10/1 -> SCOPE_PC/9
  Mux8/1 -> SCOPE_PC/6
  Mux6/1 -> SCOPE_PC/7
  Mux5/1 -> SCOPE_PC/5
  Mux7/1 -> SCOPE_PC/4
  [MR3] -> Mux11/1
  [U4] -> Mux8/2
  Mux11/1 -> SCOPE_PC/10
  [Y8_REF] -> Mux9/1
  [Y4_REF] -> Mux7/1
  [Y3_C] -> Mux4/2
  [Y4_C] -> Mux7/2
  [U1] -> Mux5/1
  Mux9/1 -> SCOPE_PC/8
  [Y1_C] -> Mux3/2
  [U3] -> Mux8/1
  [U2] -> Mux5/2
  [Y2_C] -> Mux1/2
  [Y2_REF] -> Mux1/1
  Mux3/1 -> SCOPE_PC/1
  [Y1_REF] -> Mux3/1
  [MR2] -> Mux10/2
  Mux4/1 -> Gain1/1
  Mux1/1 -> SCOPE_PC/2
  [Y3_REF] -> Mux4/1
  [Y6_REF] -> Mux6/1
  [Y7_C] -> Mux6/4
  Data Store Read2/9 -> Demux/1
  Data Store Read2/10 -> Demux1/1
  Data Store Read2/11 -> Demux2/1
  Data Store Read2/12 -> Demux3/1
  Data Store Read2/13 -> Demux4/1
  Data Store Read2/14 -> Demux5/1
  Bus Selector2/15 -> Display11/1  "<COMM_MODE>"
  Bus Selector2/16 -> Display12/1  "<UART_MODE>"
  Bus Selector2/17 -> Display13/1  "<BATTERY_VOLT>"
  Data Store Read2/17 -> [BATT_VOLT]
  [BATT_VOLT] -> Mux5/3
  [U3_R] -> Mux8/3
  [U4_R] -> Mux8/4
  [U1_R] -> Mux5/4
  [U2_R] -> Mux5/5
  ACCELERATION RATE1/1(REAL MOTOR VOLT) -> Demux6/1, Data Store Write2/1
  Demux7/1 -> [U3_R]
  Demux7/2 -> [U4_R]
  Demux6/2 -> [U2_R]
  Demux6/1 -> [U1_R]
  ACCELERATION RATE1/2(REAL MOTOR VOLT_CD) -> Demux7/1, Data Store Write3/1
  Data Store Read6/1 -> Display15/1
  Data Store Read2/20 -> [PA]
  Data Store Read2/19 -> [PA_REF]
  Data Store Read2/18 -> [PR]
  Mux2/1 -> Gain2/1
  [PA] -> Mux2/2
  [PA_REF] -> Mux2/1
  Gain2/1 -> SCOPE_PC/12
  [PR] -> Convert 2-D to 1-D/1
  Bus Selector2/4 -> Display14/1  "<CONTROL_MODE>"
  Bus Selector2/5 -> Display3/1  "<FORWARD_VEL_CONTROL_TYPE>"
  Bus Selector2/6 -> Display4/1  "<YAW_RATE_CONTROL_TYPE>"
  Bus Selector2/7 -> Display8/1  "<YAW_ANG_CONTROL_TYPE>"
  Bus Selector2/8 -> Display9/1  "<WFL_CONTROL_TYPE>"
  Bus Selector2/9 -> Display10/1  "<PITCH_ANG_CONTROL_TYPE>"
  Bus Selector2/3 -> Display16/1  "<VEHICLE_MODE>"
  [Y9_REF] -> Mux9/2
  [Y8_C] -> Mux9/3
  [Y9_C] -> Mux9/4
  [Y7_REF] -> Mux6/2
  [Y6_C] -> Mux6/3
  Convert 2-D to 1-D/1 -> SCOPE_PC/11
  Bus Selector2/1 -> Display17/1  "<MCS_RX_STATUS>"
  Data Store Read11/1 -> ACCELERATION RATE1/2(MOTOR VOLT MAX)
  Data Store Read7/1 -> ACCELERATION RATE1/1(CONTROL MOTOR VOLT)
  Bus Selector2/2 -> Display18/1  "<NAV_RX_STATUS>"

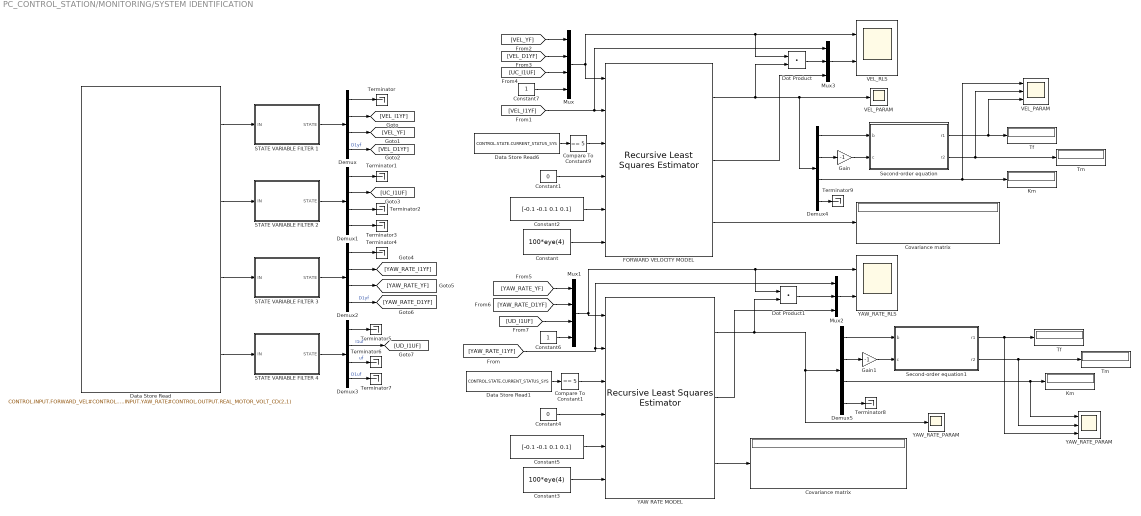
== system PC_CONTROL_STATION/MONITORING/SYSTEM IDENTIFICATION ==
  Compare To Constant1 : simulink/Logic and Bit Operations/Compare To Constant  relop===  const=5  OutDataTypeStr=boolean
  Compare To Constant9 : simulink/Logic and Bit Operations/Compare To Constant  relop===  const=5  OutDataTypeStr=boolean
  Constant : Constant  Value=100*eye(4)  SampleTime=SAMPLING_TIME
  Constant1 : Constant  Value=0  SampleTime=SAMPLING_TIME
  Constant2 : Constant  Value=[-0.1 -0.1 0.1 0.1]  SampleTime=SAMPLING_TIME
  Constant3 : Constant  Value=100*eye(4)  SampleTime=SAMPLING_TIME
  Constant4 : Constant  Value=0  SampleTime=SAMPLING_TIME
  Constant5 : Constant  Value=[-0.1 -0.1 0.1 0.1]  SampleTime=SAMPLING_TIME
  Constant6 : Constant  OutDataTypeStr=double  SampleTime=SAMPLING_TIME
  Constant7 : Constant  OutDataTypeStr=double  SampleTime=SAMPLING_TIME
  Covariance matrix : Display
  "Covariance matrix " : Display
  Data Store Read : DataStoreRead  DataStoreName=CONTROL  SampleTime=SAMPLING_TIME  DataStoreElements=CONTROL.INPUT.FORWARD_VEL#CONTROL.OUTPUT.REAL_MOTOR_VOLT_CD(1,1)#CONTROL.INPUT.YAW_RATE#CONTROL.OUTPUT.REAL_MOTOR_VOLT_CD(2,1)  IndexOptions=Index vector (dialog)  Indices=1  OutputSizes=1
  Data Store Read1 : DataStoreRead  DataStoreName=CONTROL  SampleTime=SAMPLING_TIME  DataStoreElements=CONTROL.STATE.CURRENT_STATUS_SYS  IndexOptions=Index vector (dialog)  Indices=1  OutputSizes=1
  Data Store Read6 : DataStoreRead  DataStoreName=CONTROL  SampleTime=SAMPLING_TIME  DataStoreElements=CONTROL.STATE.CURRENT_STATUS_SYS  IndexOptions=Index vector (dialog)  Indices=1  OutputSizes=1
  Demux{,1..5} (6 alike) : Demux
  Dot Product : DotProduct  OutDataTypeStr=Inherit: Inherit via internal rule
  Dot Product1 : DotProduct  OutDataTypeStr=Inherit: Inherit via internal rule
  FORWARD VELOCITY MODEL : ctrlSharedLib/Recursive Least Squares Estimator  InitialEstimateSource=External  InitialParameterData=4  P0=1e4  InitialRegressors=0  InitialOutputs=0  History=Infinite  WindowLength=200  EstimationMethod=Forgetting Factor  AdaptationParameter=0.999  HasTimeVaryingAdaptationParameter=off  NormalizationBias=eps  OutputError=on  OutputP=on  AddEnablePort=on  ExternalReset=Rising  InputProcessing=Sample-based  Ts=SAMPLING_TIME
  Gain : Gain  Gain=-1
  Gain1 : Gain  Gain=-1
  Km : Display
  "Km " : Display
  Mux : Mux
  Mux1 : Mux
  Mux2 : Mux  Inputs=3
  Mux3 : Mux  Inputs=3
  STATE VARIABLE FILTER 1 : Subsystem
  STATE VARIABLE FILTER 2 : Subsystem
  STATE VARIABLE FILTER 3 : Subsystem
  STATE VARIABLE FILTER 4 : Subsystem
  Second-order equation : MATLAB Function  TreatAsAtomicUnit=on
  Second-order equation1 : MATLAB Function  TreatAsAtomicUnit=on
  Terminator{,1..9} (10 alike) : Terminator
  Tf : Display
  "Tf " : Display
  Tm : Display
  "Tm " : Display
  VEL_PARAM : Scope
  "VEL_PARAM " : Scope  NumInputPorts=3
  VEL_RLS : Scope  NumInputPorts=2
  YAW RATE MODEL : ctrlSharedLib/Recursive Least Squares Estimator  InitialEstimateSource=External  InitialParameterData=4  P0=1e4  InitialRegressors=0  InitialOutputs=0  History=Infinite  WindowLength=200  EstimationMethod=Forgetting Factor  AdaptationParameter=0.999  HasTimeVaryingAdaptationParameter=off  NormalizationBias=eps  OutputError=on  OutputP=on  AddEnablePort=on  ExternalReset=Rising  InputProcessing=Sample-based  Ts=SAMPLING_TIME
  YAW_RATE_PARAM : Scope
  "YAW_RATE_PARAM " : Scope  NumInputPorts=3
  YAW_RATE_RLS : Scope  NumInputPorts=2
  wires:
  STATE VARIABLE FILTER 1/1(STATE) -> Demux/1
  Demux/1 -> Terminator/1
  STATE VARIABLE FILTER 2/1(STATE) -> Demux1/1
  Demux1/1 -> Terminator1/1
  Demux1/3 -> Terminator2/1
  Demux1/4 -> Terminator3/1
  Constant/1 -> FORWARD VELOCITY MODEL/6
  Constant1/1 -> FORWARD VELOCITY MODEL/4
  Constant2/1 -> FORWARD VELOCITY MODEL/5
  Constant5/1 -> YAW RATE MODEL/5
  Constant4/1 -> YAW RATE MODEL/4
  Constant3/1 -> YAW RATE MODEL/6
  Mux1/1 -> Dot Product1/1, YAW_RATE_RLS/1, YAW RATE MODEL/1
  STATE VARIABLE FILTER 3/1(STATE) -> Demux2/1
  STATE VARIABLE FILTER 4/1(STATE) -> Demux3/1
  Demux2/1 -> Terminator4/1
  Demux3/1 -> Terminator5/1
  Demux3/3 -> Terminator6/1  "uf"
  Demux3/4 -> Terminator7/1  "D1uf"
  Demux4/3 -> "VEL_PARAM "/1, Km/1
  Second-order equation/1(r1) -> "VEL_PARAM "/3, Tf/1
  Second-order equation/2(r2) -> "VEL_PARAM "/2, Tm/1
  YAW RATE MODEL/1 -> Dot Product1/2, YAW_RATE_PARAM/1, Demux5/1
  Data Store Read/1 -> STATE VARIABLE FILTER 1/1(IN)
  Data Store Read/2 -> STATE VARIABLE FILTER 2/1(IN)
  Data Store Read/4 -> STATE VARIABLE FILTER 4/1(IN)
  Data Store Read/3 -> STATE VARIABLE FILTER 3/1(IN)
  Demux/2 -> [VEL_I1YF]
  Demux/3 -> [VEL_YF]
  Demux/4 -> [VEL_D1YF]  "D1yf"
  Demux1/2 -> [UC_I1UF]
  [UC_I1UF] -> Mux/3
  Demux2/2 -> [YAW_RATE_I1YF]
  [YAW_RATE_I1YF] -> Mux2/1, YAW RATE MODEL/2
  Demux2/3 -> [YAW_RATE_YF]
  Demux2/4 -> [YAW_RATE_D1YF]  "D1yf"
  Demux3/2 -> [UD_I1UF]  "I1uf"
  [UD_I1UF] -> Mux1/3
  [VEL_D1YF] -> Mux/2
  [VEL_YF] -> Mux/1
  [YAW_RATE_D1YF] -> Mux1/2
  [YAW_RATE_YF] -> Mux1/1
  Demux4/2 -> Gain/1
  Gain/1 -> Second-order equation/2(c)
  Demux4/1 -> Second-order equation/1(b)
  Demux5/2 -> Gain1/1
  Gain1/1 -> Second-order equation1/2(c)
  Demux5/1 -> Second-order equation1/1(b)
  FORWARD VELOCITY MODEL/3 -> Covariance matrix/1
  YAW RATE MODEL/3 -> "Covariance matrix "/1
  Compare To Constant1/1 -> YAW RATE MODEL/3
  YAW RATE MODEL/2 -> Mux2/3
  Mux2/1 -> YAW_RATE_RLS/2
  Dot Product1/1 -> Mux2/2
  Dot Product/1 -> Mux3/2
  Mux3/1 -> VEL_RLS/2
  FORWARD VELOCITY MODEL/2 -> Mux3/3
  [VEL_I1YF] -> Mux3/1, FORWARD VELOCITY MODEL/2
  FORWARD VELOCITY MODEL/1 -> Dot Product/2, VEL_PARAM/1, Demux4/1
  Mux/1 -> FORWARD VELOCITY MODEL/1, Dot Product/1, VEL_RLS/1
  Demux5/3 -> "YAW_RATE_PARAM "/1, "Km "/1
  Second-order equation1/2(r2) -> "YAW_RATE_PARAM "/2, "Tm "/1
  Second-order equation1/1(r1) -> "YAW_RATE_PARAM "/3, "Tf "/1
  Constant6/1 -> Mux1/4
  Demux5/4 -> Terminator8/1
  Demux4/4 -> Terminator9/1
  Constant7/1 -> Mux/4
  Compare To Constant9/1 -> FORWARD VELOCITY MODEL/3
  Data Store Read6/1 -> Compare To Constant9/1
  Data Store Read1/1 -> Compare To Constant1/1

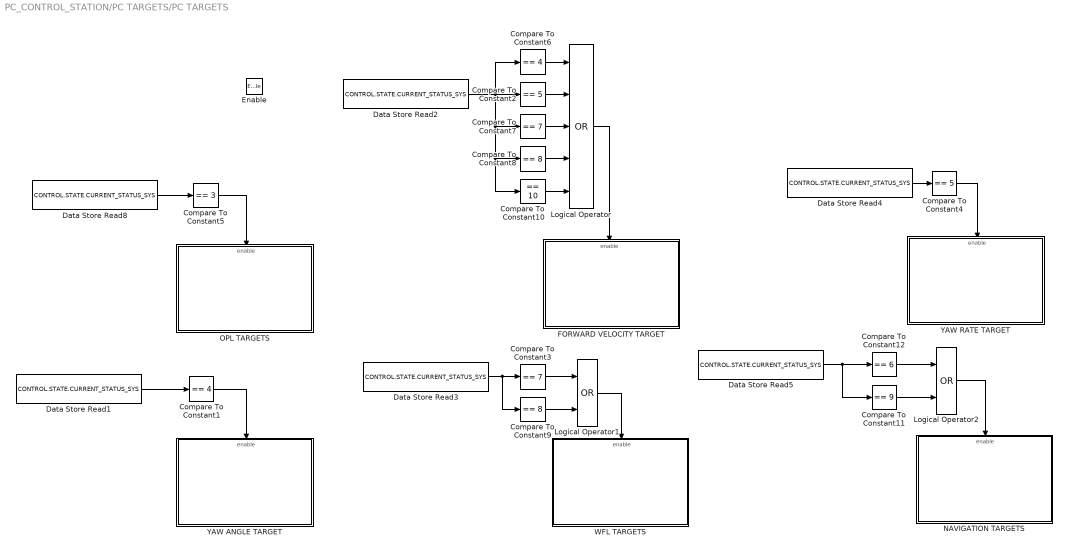
== system PC_CONTROL_STATION/PC TARGETS/PC TARGETS ==
  Enable : EnablePort
  Compare To Constant1 : simulink/Logic and Bit Operations/Compare To Constant  relop===  const=4  OutDataTypeStr=boolean
  Compare To Constant10 : simulink/Logic and Bit Operations/Compare To Constant  relop===  const=10  OutDataTypeStr=boolean
  Compare To Constant11 : simulink/Logic and Bit Operations/Compare To Constant  relop===  const=9  OutDataTypeStr=boolean
  Compare To Constant12 : simulink/Logic and Bit Operations/Compare To Constant  relop===  const=6  OutDataTypeStr=boolean
  Compare To Constant2 : simulink/Logic and Bit Operations/Compare To Constant  relop===  const=5  OutDataTypeStr=boolean
  Compare To Constant3 : simulink/Logic and Bit Operations/Compare To Constant  relop===  const=7  OutDataTypeStr=boolean
  Compare To Constant4 : simulink/Logic and Bit Operations/Compare To Constant  relop===  const=5  OutDataTypeStr=boolean
  Compare To Constant5 : simulink/Logic and Bit Operations/Compare To Constant  relop===  const=3  OutDataTypeStr=boolean
  Compare To Constant6 : simulink/Logic and Bit Operations/Compare To Constant  relop===  const=4  OutDataTypeStr=boolean
  Compare To Constant7 : simulink/Logic and Bit Operations/Compare To Constant  relop===  const=7  OutDataTypeStr=boolean
  Compare To Constant8 : simulink/Logic and Bit Operations/Compare To Constant  relop===  const=8  OutDataTypeStr=boolean
  Compare To Constant9 : simulink/Logic and Bit Operations/Compare To Constant  relop===  const=8  OutDataTypeStr=boolean
  Data Store Read{1..5,8} (6 alike) : DataStoreRead  DataStoreName=CONTROL  SampleTime=SAMPLING_TIME  DataStoreElements=CONTROL.STATE.CURRENT_STATUS_SYS  IndexOptions=Index vector (dialog)  Indices=1  OutputSizes=1
  FORWARD VELOCITY TARGET : Subsystem
  Logical Operator : Logic  Operator=OR  Inputs=5  AllPortsSameDT=off  OutDataTypeStr=boolean
  Logical Operator1 : Logic  Operator=OR  AllPortsSameDT=off  OutDataTypeStr=boolean
  Logical Operator2 : Logic  Operator=OR  AllPortsSameDT=off  OutDataTypeStr=boolean
  NAVIGATION TARGETS : Subsystem  Priority=10
      settings: MinAlgLoopOccurrences=on
  OPL TARGETS : Subsystem
  WFL TARGETS : Subsystem
  YAW ANGLE TARGET : Subsystem
  YAW RATE TARGET : Subsystem
  wires:
  Compare To Constant5/1 -> OPL TARGETS/Enable
  Data Store Read8/1 -> Compare To Constant5/1
  Data Store Read2/1 -> Compare To Constant10/1, Compare To Constant8/1, Compare To Constant7/1, Compare To Constant6/1, Compare To Constant2/1
  Data Store Read3/1 -> Compare To Constant9/1, Compare To Constant3/1
  Data Store Read4/1 -> Compare To Constant4/1
  Compare To Constant4/1 -> YAW RATE TARGET/Enable
  Compare To Constant6/1 -> Logical Operator/1
  Compare To Constant2/1 -> Logical Operator/2
  Logical Operator/1 -> FORWARD VELOCITY TARGET/Enable
  Compare To Constant7/1 -> Logical Operator/3
  Compare To Constant8/1 -> Logical Operator/4
  Logical Operator1/1 -> WFL TARGETS/Enable
  Compare To Constant3/1 -> Logical Operator1/1
  Compare To Constant9/1 -> Logical Operator1/2
  Compare To Constant10/1 -> Logical Operator/5
  Compare To Constant1/1 -> YAW ANGLE TARGET/Enable
  Data Store Read1/1 -> Compare To Constant1/1
  Logical Operator2/1 -> NAVIGATION TARGETS/Enable
  Compare To Constant11/1 -> Logical Operator2/2
  Compare To Constant12/1 -> Logical Operator2/1
  Data Store Read5/1 -> Compare To Constant11/1, Compare To Constant12/1

== system PC_CONTROL_STATION/HARDWARE/ROS2_MONITORING/MSG_RX ==
  Bus Assignment : BusAssignment  AssignedSignals=RX_BUFFER
  Bus Selector : BusSelector  OutputSignals=data
  Constant : Constant  Commented=on  Value=zeros(1,1400,'uint8')  SampleTime=CONTROL_INI.PARAM.COMM_SAMPLING_TIME
  Data Store Read : DataStoreRead  DataStoreName=MSG  IndexOptions=Index vector (dialog)  Indices=1  OutputSizes=1
  Data Store Write1 : DataStoreWrite  DataStoreName=MSG  IndexOptions=Index vector (dialog)  Indices=1  OutputSizes=1
  Subscribe : ros2lib/Subscribe  topicSource=Specify your own  topic=/car_to_pc  messageType=std_msgs/UInt8MultiArray  sampleTime=CONTROL_INI.PARAM.COMM_SAMPLING_TIME  QOSHistory=Keep last  QOSDepth=1  QOSReliability=Best effort  QOSDurability=Volatile
  Terminator : Terminator
  wires:
  Data Store Read/1 -> Bus Assignment/1
  Bus Assignment/1 -> Data Store Write1/1
  Subscribe/2 -> Bus Selector/1
  Bus Selector/1 -> Bus Assignment/2  "<data>"
  Subscribe/1 -> Terminator/1

== system PC_CONTROL_STATION/HARDWARE/ROS2_MONITORING/MSG_TX  ==
  Enable : EnablePort
  Blank Message : ros2lib/Blank Message  messageClass=Message  entityType=std_msgs/UInt8MultiArray  messageType=std_msgs/UInt8MultiArray  SampleTime=CONTROL_INI.PARAM.COMM_SAMPLING_TIME
  Bus Assignment : BusAssignment  AssignedSignals=data,data_SL_Info.CurrentLength
  Constant : Constant  Value=1400  OutDataTypeStr=uint32  SampleTime=CONTROL_INI.PARAM.COMM_SAMPLING_TIME
  Data Store Read1 : DataStoreRead  DataStoreName=MSG  SampleTime=CONTROL_INI.PARAM.COMM_SAMPLING_TIME  DataStoreElements=MSG.TX_BUFFER(:,1)  IndexOptions=Index vector (dialog)  Indices=1  OutputSizes=1
  Publish : ros2lib/Publish  topicSource=Specify your own  topic=/pc_to_car  messageType=std_msgs/UInt8MultiArray  QOSHistory=Keep last  QOSDepth=1  QOSReliability=Best effort  QOSDurability=Volatile
  wires:
  Data Store Read1/1 -> Bus Assignment/2
  Bus Assignment/1 -> Publish/1
  Blank Message/1 -> Bus Assignment/1
  Constant/1 -> Bus Assignment/3

== system PC_CONTROL_STATION/HARDWARE/RT_MONITORING/TCP 101 ==
  Compare To Zero : simulink/Logic and Bit Operations/Compare To Zero  relop=>  OutDataTypeStr=boolean
  Data Store Read : DataStoreRead  DataStoreName=MSG  SampleTime=CONTROL_INI.PARAM.COMM_SAMPLING_TIME  DataStoreElements=MSG.TX_BUFFER(1,1)  IndexOptions=Index vector (dialog)  Indices=1  OutputSizes=1
  MSG_RX : Subsystem  Priority=10
      settings: RTWSystemCode=Nonreusable function  FunctionWithSeparateData=on
  "MSG_TX " : Subsystem  Priority=10
      settings: RTWSystemCode=Nonreusable function  FunctionWithSeparateData=on
  wires:
  Compare To Zero/1 -> "MSG_TX "/Enable
  Data Store Read/1 -> Compare To Zero/1

== system PC_CONTROL_STATION/HARDWARE/RT_MONITORING/TCP 102 ==
  Compare To Zero : simulink/Logic and Bit Operations/Compare To Zero  relop=>  OutDataTypeStr=boolean
  Data Store Read : DataStoreRead  DataStoreName=MSG  SampleTime=CONTROL_INI.PARAM.COMM_SAMPLING_TIME  DataStoreElements=MSG.TX_BUFFER(1,1)  IndexOptions=Index vector (dialog)  Indices=1  OutputSizes=1
  MSG_RX : Subsystem  Priority=10
      settings: RTWSystemCode=Nonreusable function  FunctionWithSeparateData=on
  "MSG_TX " : Subsystem  Priority=10
      settings: RTWSystemCode=Nonreusable function  FunctionWithSeparateData=on
  wires:
  Compare To Zero/1 -> "MSG_TX "/Enable
  Data Store Read/1 -> Compare To Zero/1

== system PC_CONTROL_STATION/HARDWARE/RT_MONITORING/TCP 103 ==
  Compare To Zero : simulink/Logic and Bit Operations/Compare To Zero  relop=>  OutDataTypeStr=boolean
  Data Store Read : DataStoreRead  DataStoreName=MSG  SampleTime=CONTROL_INI.PARAM.COMM_SAMPLING_TIME  DataStoreElements=MSG.TX_BUFFER(1,1)  IndexOptions=Index vector (dialog)  Indices=1  OutputSizes=1
  MSG_RX : Subsystem  Priority=10
      settings: RTWSystemCode=Nonreusable function  FunctionWithSeparateData=on
  "MSG_TX " : Subsystem  Priority=10
      settings: RTWSystemCode=Nonreusable function  FunctionWithSeparateData=on
  wires:
  Compare To Zero/1 -> "MSG_TX "/Enable
  Data Store Read/1 -> Compare To Zero/1

== system PC_CONTROL_STATION/HARDWARE/RT_MONITORING/TCP 104 ==
  Compare To Zero : simulink/Logic and Bit Operations/Compare To Zero  relop=>  OutDataTypeStr=boolean
  Data Store Read : DataStoreRead  DataStoreName=MSG  SampleTime=CONTROL_INI.PARAM.COMM_SAMPLING_TIME  DataStoreElements=MSG.TX_BUFFER(1,1)  IndexOptions=Index vector (dialog)  Indices=1  OutputSizes=1
  MSG_RX : Subsystem  Priority=10
      settings: RTWSystemCode=Nonreusable function  FunctionWithSeparateData=on
  "MSG_TX " : Subsystem  Priority=10
      settings: RTWSystemCode=Nonreusable function  FunctionWithSeparateData=on
  wires:
  Compare To Zero/1 -> "MSG_TX "/Enable
  Data Store Read/1 -> Compare To Zero/1

== system PC_CONTROL_STATION/HARDWARE/RT_MONITORING/TCP 105 ==
  Compare To Zero : simulink/Logic and Bit Operations/Compare To Zero  relop=>  OutDataTypeStr=boolean
  Data Store Read : DataStoreRead  DataStoreName=MSG  SampleTime=CONTROL_INI.PARAM.COMM_SAMPLING_TIME  DataStoreElements=MSG.TX_BUFFER(1,1)  IndexOptions=Index vector (dialog)  Indices=1  OutputSizes=1
  MSG_RX : Subsystem  Priority=10
      settings: RTWSystemCode=Nonreusable function  FunctionWithSeparateData=on
  "MSG_TX " : Subsystem  Priority=10
      settings: RTWSystemCode=Nonreusable function  FunctionWithSeparateData=on
  wires:
  Compare To Zero/1 -> "MSG_TX "/Enable
  Data Store Read/1 -> Compare To Zero/1
